simulink model "PassiveHydPTO_Version_2"  (R2014a)
settings: Solver=ode23tb  StartTime=0.0  StopTime=param.stop  FixedStep=0.01  MaxStep=0.05  RelTol=1e-6
values from neighbouring files (symbols this model uses):
  alpha = 1    [Main.m]
  Amax = 0.001    [Main.m]
  Amin = 1e-8    (= 1e-08)    [Main.m]
  Ap = 2.35e-2    (= 0.0235)    [Main.m]
  Beta_e = 1.86e9    (= 1860000000)    [Main.m]
  bf = 0.05*bg    (= 0.118735)    [Main.m]
  bg = 2.3747    [Main.m]
  Cd = 0.61    [Main.m]
  D = 3.9789e-5    (= 3.9789e-05)    [Main.m]
  Dh = sqrt(4*Av/pi)    [Main.m]
  f = 1/period    (= 0.1)    [Main.m]
  J = 3.961    [Main.m]
  k1 = 200    [Main.m]
  k2 = atanh((Amin-(Amax-Amin)/2)*      2/(Amax - Amin))*1/(pMin-(pMax + pMin)/2)    [Main.m]
  omega_i = 0    [Main.m]
  pAeq = pCeq    (= 21333333.3333)    [Main.m]
  pAi = pAeq    (= 21333333.3333)    [Main.m]
  pAupper_limit = 32e6    (= 32000000)    [Main.m]
  pBeq = pCeq    (= 21333333.3333)    [Main.m]
  pBi = pBeq    (= 21333333.3333)    [Main.m]
  pBupper_limit = 32e6    (= 32000000)    [Main.m]
  pCprecharge = 0.9*pClower_limit    (= 19200000)    [Main.m]
  pDprecharge = 0.9*pDlower_limit    (= 9600000)    [Main.m]
  pMax = 1e6    (= 1000000)    [Main.m]
  pMin = 0.75e6    (= 750000)    [Main.m]
  rho = 850    [Main.m]
  Rt = 10    [Main.m]
  v = 5.5e-5    (= 5.5e-05)    [Main.m]
  VC0 = 7.5    [Main.m]
  VCeq = VC0*(1-(pCprecharge/pCeq)^(1/1.4))    (= 0.543715404282)    [Main.m]
  VD0 = 3    [Main.m]
  VDeq = VDmax    (= 1.30403881906)    [Main.m]
  Vo = Ap*5    (= 0.1175)    [Main.m]
undefined symbols (not defined in the file or in its folder): magnitude
settings Model: Creator=sor  LastModifiedBy=sor

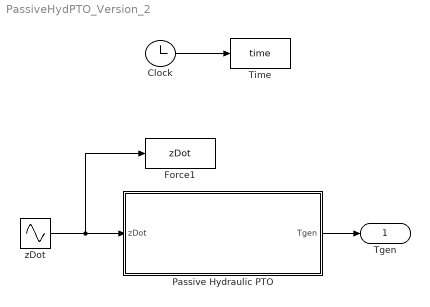
== system PassiveHydPTO_Version_2 ==
  Clock : Clock
  Force1 : ToWorkspace  VariableName=zDot  SampleTime=-1
  "Passive Hydraulic PTO " : Subsystem
  Time : ToWorkspace  VariableName=time  SampleTime=-1
  zDot : Sin  Amplitude=0.8  Frequency=2*pi*f  SampleTime=0
  Tgen : Outport
  wires:
  Clock/1 -> Time/1
  zDot/1 -> Force1/1, "Passive Hydraulic PTO "/1(zDot)
  "Passive Hydraulic PTO "/1(Tgen) -> Tgen/1

== system PassiveHydPTO_Version_2/Passive Hydraulic PTO  ==
  zDot : Inport
  High Pressure Accumulator : Subsystem
  Low Pressure Accumulator : Subsystem
  Motor Generator : Subsystem
  "Piston Pump " : Subsystem
  Rectified Valve : Subsystem
  Tgen : Outport
  wires:
  "Piston Pump "/1(pA) -> Rectified Valve/1(pA)
  Motor Generator/1(Tgen) -> Tgen/1
  Rectified Valve/1(Vdot1) -> High Pressure Accumulator/1(Vdot1)
  Rectified Valve/2(Vdot2) -> High Pressure Accumulator/2(Vdot2)
  Rectified Valve/3(Vdot3) -> Low Pressure Accumulator/1(Vdot3)
  Rectified Valve/4(Vdot4) -> Low Pressure Accumulator/2(Vdot4)
  High Pressure Accumulator/1(pC) -> Motor Generator/1(pC)
  Low Pressure Accumulator/1(pD) -> Motor Generator/2(pD)
  "Piston Pump "/2(pB) -> Rectified Valve/2(pB)
  zDot/1 -> "Piston Pump "/1(zDot)

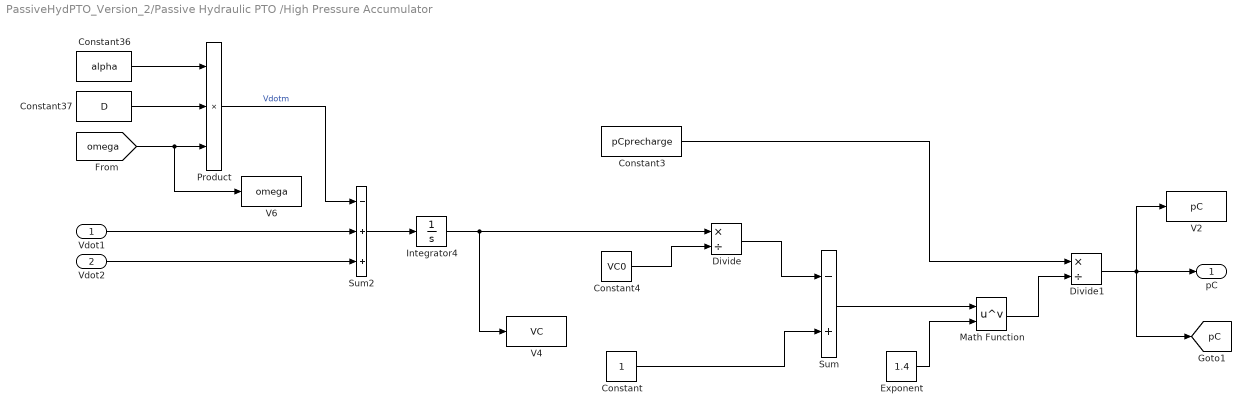
== system PassiveHydPTO_Version_2/Passive Hydraulic PTO /High Pressure Accumulator ==
  Vdot1 : Inport
  Vdot2 : Inport  Port=2
  Constant : Constant
  Constant3 : Constant  Value=pCprecharge
  Constant36 : Constant  Value=alpha
  Constant37 : Constant  Value=D
  Constant4 : Constant  Value=VC0
  Divide : Product  Inputs=*/
  Divide1 : Product  Inputs=*/
  Exponent : Constant  Value=1.4
  Integrator4 : Integrator  InitialCondition=VCeq
  Math Function : Math  Operator=pow  SaturateOnIntegerOverflow=on
  Product : Product  Inputs=3
  Sum : Sum  Inputs=-+
  Sum2 : Sum  Inputs=-++
  V2 : ToWorkspace  VariableName=pC  SampleTime=-1
  V4 : ToWorkspace  VariableName=VC  SampleTime=-1
  V6 : ToWorkspace  VariableName=omega  SampleTime=-1
  pC : Outport
  tag scope: pC=global
  wires:
  Constant36/1 -> Product/1
  Constant37/1 -> Product/2
  [omega] -> V6/1, Product/3
  Product/1 -> Sum2/1  "Vdotm"
  Vdot1/1 -> Sum2/2
  Vdot2/1 -> Sum2/3
  Sum2/1 -> Integrator4/1
  Integrator4/1 -> Divide/1, V4/1
  Constant4/1 -> Divide/2
  Constant/1 -> Sum/2
  Divide/1 -> Sum/1
  Exponent/1 -> Math Function/2
  Sum/1 -> Math Function/1
  Math Function/1 -> Divide1/2
  Constant3/1 -> Divide1/1
  Divide1/1 -> [pC], V2/1, pC/1

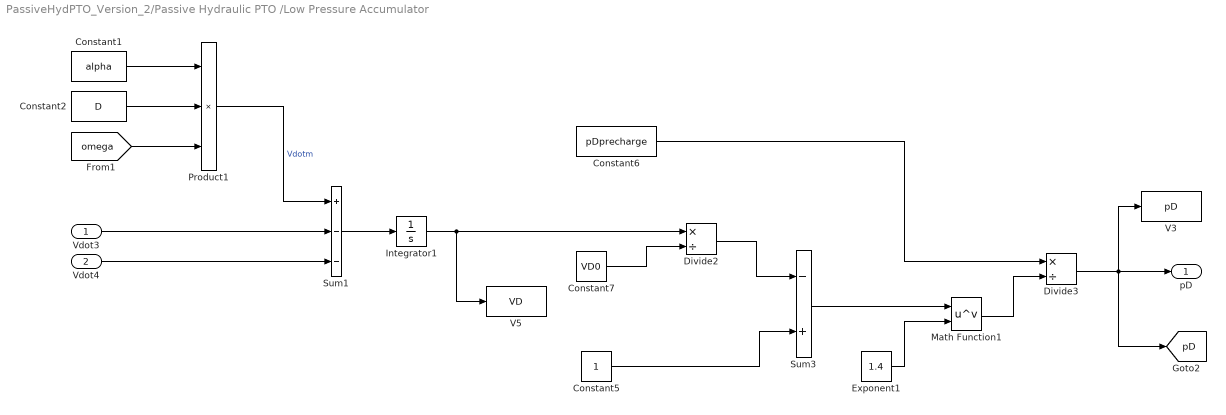
== system PassiveHydPTO_Version_2/Passive Hydraulic PTO /Low Pressure Accumulator ==
  Vdot3 : Inport
  Vdot4 : Inport  Port=2
  Constant1 : Constant  Value=alpha
  Constant2 : Constant  Value=D
  Constant5 : Constant
  Constant6 : Constant  Value=pDprecharge
  Constant7 : Constant  Value=VD0
  Divide2 : Product  Inputs=*/
  Divide3 : Product  Inputs=*/
  Exponent1 : Constant  Value=1.4
  Integrator1 : Integrator  InitialCondition=VDeq
  Math Function1 : Math  Operator=pow  SaturateOnIntegerOverflow=on
  Product1 : Product  Inputs=3
  Sum1 : Sum  Inputs=+--
  Sum3 : Sum  Inputs=-+
  V3 : ToWorkspace  VariableName=pD  SampleTime=-1
  V5 : ToWorkspace  VariableName=VD  SampleTime=-1
  pD : Outport
  tag scope: pD=global
  wires:
  Constant1/1 -> Product1/1
  Constant2/1 -> Product1/2
  [omega] -> Product1/3
  Product1/1 -> Sum1/1  "Vdotm"
  Vdot3/1 -> Sum1/2
  Vdot4/1 -> Sum1/3
  Sum1/1 -> Integrator1/1
  Integrator1/1 -> Divide2/1, V5/1
  Constant7/1 -> Divide2/2
  Constant5/1 -> Sum3/2
  Divide2/1 -> Sum3/1
  Exponent1/1 -> Math Function1/2
  Sum3/1 -> Math Function1/1
  Math Function1/1 -> Divide3/2
  Constant6/1 -> Divide3/1
  Divide3/1 -> [pD], V3/1, pD/1

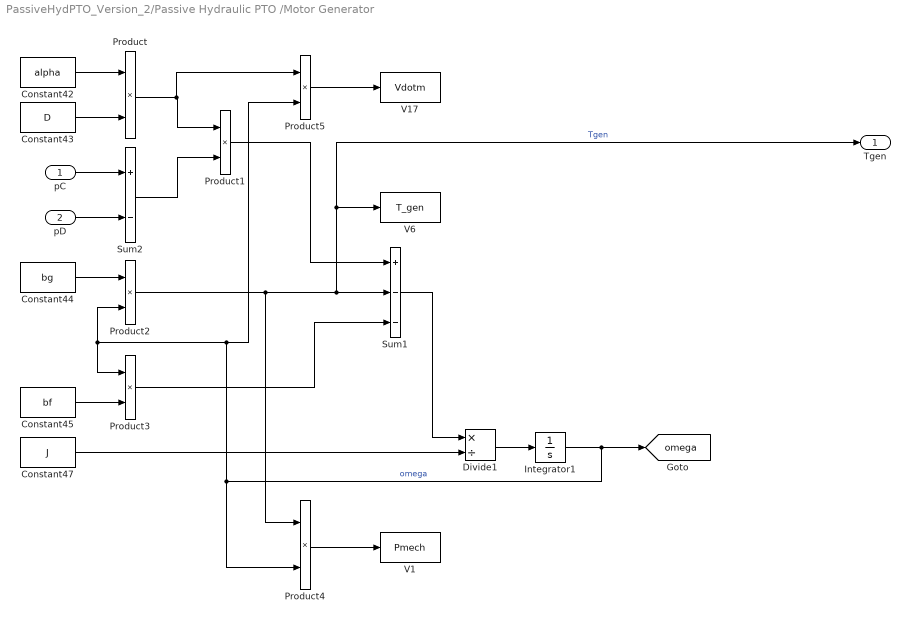
== system PassiveHydPTO_Version_2/Passive Hydraulic PTO /Motor Generator ==
  pC : Inport
  pD : Inport  Port=2
  Constant42 : Constant  Value=alpha
  Constant43 : Constant  Value=D
  Constant44 : Constant  Value=bg
  Constant45 : Constant  Value=bf
  Constant47 : Constant  Value=J
  Divide1 : Product  Inputs=*/
  Integrator1 : Integrator  InitialCondition=omega_i
  Product{,1..5} (6 alike) : Product
  Sum1 : Sum  Inputs=+--
  Sum2 : Sum  Inputs=+-
  V1 : ToWorkspace  VariableName=Pmech  SampleTime=-1
  V17 : ToWorkspace  VariableName=Vdotm  SampleTime=-1
  V6 : ToWorkspace  VariableName=T_gen  SampleTime=-1
  Tgen : Outport
  tag scope: omega=global
  wires:
  Constant42/1 -> Product/1
  Constant43/1 -> Product/2
  pC/1 -> Sum2/1
  pD/1 -> Sum2/2
  Product/1 -> Product5/1, Product1/1
  Sum2/1 -> Product1/2
  Constant44/1 -> Product2/1
  Constant45/1 -> Product3/2
  Product1/1 -> Sum1/1
  Product2/1 -> Product4/1, Tgen/1, V6/1, Sum1/2  "Tgen"
  Product3/1 -> Sum1/3
  Sum1/1 -> Divide1/1
  Constant47/1 -> Divide1/2
  Product4/1 -> V1/1
  Divide1/1 -> Integrator1/1
  Integrator1/1 -> Product4/2, Product3/1, Product2/2, Product5/2, [omega]  "omega"
  Product5/1 -> V17/1

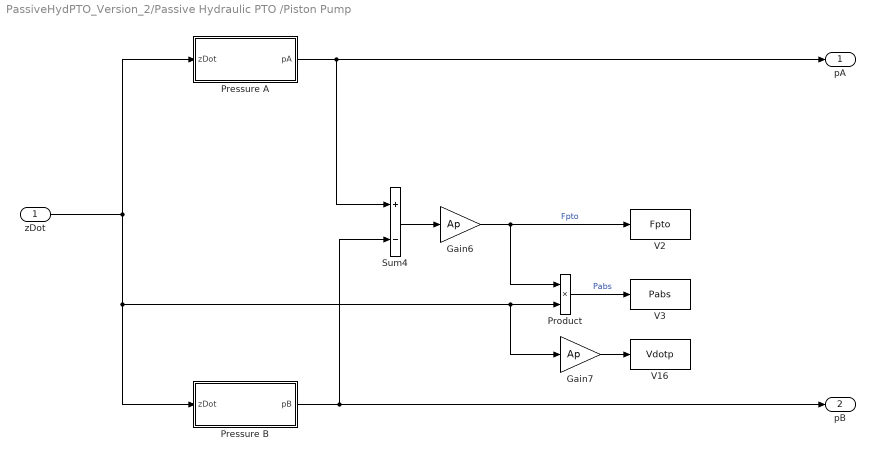
== system PassiveHydPTO_Version_2/Passive Hydraulic PTO /Piston Pump  ==
  zDot : Inport
  Gain6 : Gain  Gain=Ap
  Gain7 : Gain  Gain=Ap
  Pressure A : Subsystem
  Pressure B : Subsystem
  Product : Product
  Sum4 : Sum  Inputs=+-
  V16 : ToWorkspace  VariableName=Vdotp  SampleTime=-1
  V2 : ToWorkspace  VariableName=Fpto  SampleTime=-1
  V3 : ToWorkspace  VariableName=Pabs  SampleTime=-1
  pA : Outport
  pB : Outport  Port=2
  wires:
  zDot/1 -> Pressure A/1(zDot), Gain7/1, Product/2, Pressure B/1(zDot)
  Pressure A/1(pA) -> pA/1, Sum4/1
  Pressure B/1(pB) -> Sum4/2, pB/1
  Sum4/1 -> Gain6/1
  Gain7/1 -> V16/1
  Gain6/1 -> V2/1, Product/1  "Fpto"
  Product/1 -> V3/1  "Pabs"

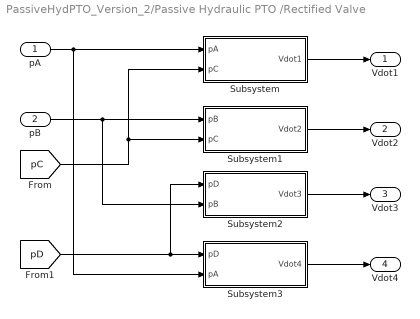
== system PassiveHydPTO_Version_2/Passive Hydraulic PTO /Rectified Valve ==
  pA : Inport
  pB : Inport  Port=2
  Subsystem : Subsystem
  Subsystem1 : Subsystem
  Subsystem2 : Subsystem
  Subsystem3 : Subsystem
  Vdot1 : Outport
  Vdot2 : Outport  Port=2
  Vdot3 : Outport  Port=3
  Vdot4 : Outport  Port=4
  wires:
  pA/1 -> Subsystem/1(pA), Subsystem3/2(pA)
  pB/1 -> Subsystem2/2(pB), Subsystem1/1(pB)
  [pC] -> Subsystem1/2(pC), Subsystem/2(pC)
  [pD] -> Subsystem3/1(pD), Subsystem2/1(pD)
  Subsystem3/1(Vdot4) -> Vdot4/1
  Subsystem2/1(Vdot3) -> Vdot3/1
  Subsystem1/1(Vdot2) -> Vdot2/1
  Subsystem/1(Vdot1) -> Vdot1/1

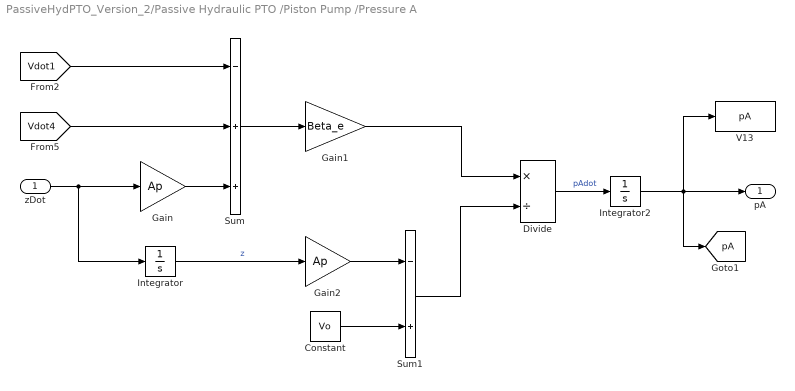
== system PassiveHydPTO_Version_2/Passive Hydraulic PTO /Piston Pump /Pressure A ==
  zDot : Inport
  Constant : Constant  Value=Vo
  Divide : Product  Inputs=*/
  Gain : Gain  Gain=Ap
  Gain1 : Gain  Gain=Beta_e
  Gain2 : Gain  Gain=Ap
  Integrator : Integrator
  Integrator2 : Integrator  InitialCondition=pAi  UpperSaturationLimit=pAupper_limit  LowerSaturationLimit=pAeq
  Sum : Sum  Inputs=-++
  Sum1 : Sum  Inputs=-+
  V13 : ToWorkspace  VariableName=pA  SampleTime=-1
  pA : Outport
  tag scope: pA=global
  wires:
  Gain/1 -> Sum/3
  Sum/1 -> Gain1/1
  zDot/1 -> Integrator/1, Gain/1
  Integrator/1 -> Gain2/1  "z"
  Gain2/1 -> Sum1/1
  Constant/1 -> Sum1/2
  Gain1/1 -> Divide/1
  Sum1/1 -> Divide/2
  [Vdot1] -> Sum/1
  Divide/1 -> Integrator2/1  "pAdot"
  [Vdot4] -> Sum/2
  Integrator2/1 -> pA/1, [pA], V13/1

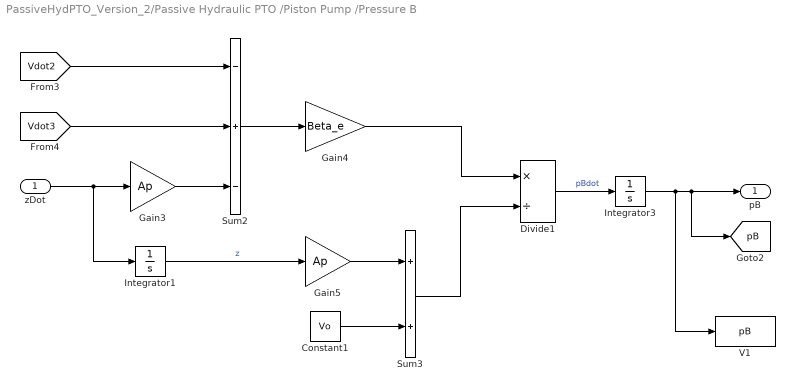
== system PassiveHydPTO_Version_2/Passive Hydraulic PTO /Piston Pump /Pressure B ==
  zDot : Inport
  Constant1 : Constant  Value=Vo
  Divide1 : Product  Inputs=*/
  Gain3 : Gain  Gain=Ap
  Gain4 : Gain  Gain=Beta_e
  Gain5 : Gain  Gain=Ap
  Integrator1 : Integrator
  Integrator3 : Integrator  InitialCondition=pBi  UpperSaturationLimit=pBupper_limit  LowerSaturationLimit=pBeq
  Sum2 : Sum  Inputs=-+-
  Sum3 : Sum
  V1 : ToWorkspace  VariableName=pB  SampleTime=-1
  pB : Outport
  tag scope: pB=global
  wires:
  Gain3/1 -> Sum2/3
  Sum2/1 -> Gain4/1
  zDot/1 -> Integrator1/1, Gain3/1
  Integrator1/1 -> Gain5/1  "z"
  Gain5/1 -> Sum3/1
  Constant1/1 -> Sum3/2
  Gain4/1 -> Divide1/1
  Sum3/1 -> Divide1/2
  Divide1/1 -> Integrator3/1  "pBdot"
  [Vdot2] -> Sum2/1
  [Vdot3] -> Sum2/2
  Integrator3/1 -> V1/1, pB/1, [pB]

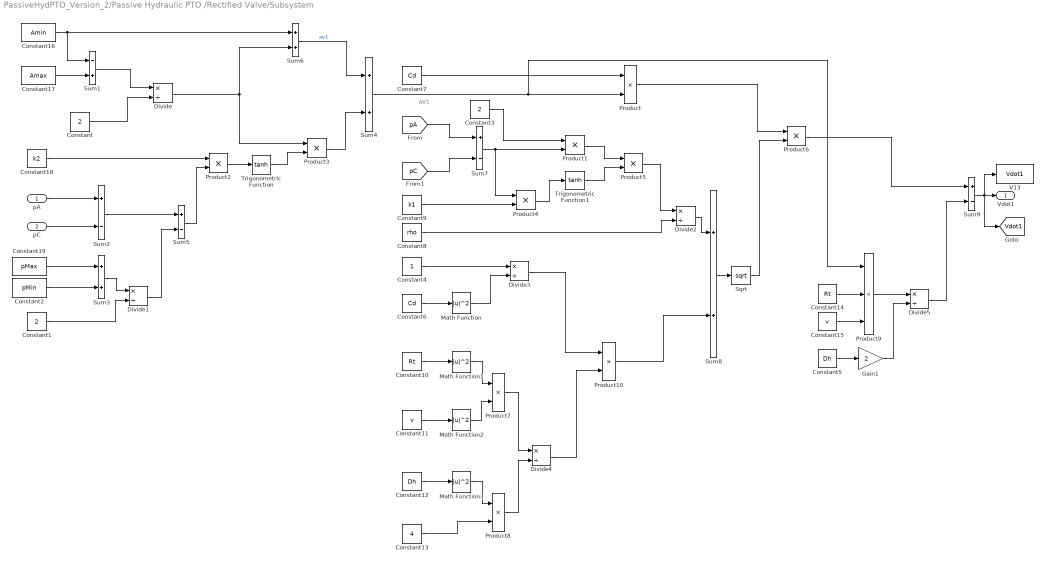
== system PassiveHydPTO_Version_2/Passive Hydraulic PTO /Rectified Valve/Subsystem ==
  note: aV1
  pA : Inport
  pC : Inport  Port=2
  Constant : Constant  Value=2
  Constant1 : Constant  Value=2
  Constant10 : Constant  Value=Rt
  Constant11 : Constant  Value=v
  Constant12 : Constant  Value=Dh
  Constant13 : Constant  Value=4
  Constant14 : Constant  Value=Rt
  Constant15 : Constant  Value=v
  Constant16 : Constant  Value=Amin
  Constant17 : Constant  Value=Amax
  Constant18 : Constant  Value=k2
  Constant19 : Constant  Value=pMax
  Constant2 : Constant  Value=pMin
  Constant3 : Constant  Value=2
  Constant4 : Constant
  Constant5 : Constant  Value=Dh
  Constant6 : Constant  Value=Cd
  Constant7 : Constant  Value=Cd
  Constant8 : Constant  Value=rho
  Constant9 : Constant  Value=k1
  Divide{,1..5} (6 alike) : Product  Inputs=*/
  Gain1 : Gain  Gain=2
  Math Function{,1..3} (4 alike) : Math  Operator=magnitude^2  SaturateOnIntegerOverflow=on
  Product{,1..8,10} (10 alike) : Product
  Product9 : Product  Inputs=3
  Sqrt : Sqrt  SaturateOnIntegerOverflow=on
  Sum1 : Sum  Inputs=-+
  Sum{2,5,7,9} (4 alike) : Sum  Inputs=+-
  Sum{3..4,6,8} (4 alike) : Sum
  Trigonometric Function : Trigonometry  Operator=tanh
  Trigonometric Function1 : Trigonometry  Operator=tanh
  V13 : ToWorkspace  VariableName=Vdot1  SampleTime=-1
  Vdot1 : Outport
  tag scope: Vdot1=global
  wires:
  Constant16/1 -> Sum6/1, Sum1/1
  Constant17/1 -> Sum1/2
  Sum1/1 -> Divide/1
  Constant/1 -> Divide/2
  Product2/1 -> Trigonometric Function/1
  Trigonometric Function/1 -> Product3/2
  Product3/1 -> Sum4/2
  pA/1 -> Sum2/1
  Constant19/1 -> Sum3/1
  Constant2/1 -> Sum3/2
  Sum3/1 -> Divide1/1
  Constant1/1 -> Divide1/2
  Divide/1 -> Sum6/2, Product3/1
  Sum2/1 -> Sum5/1
  Divide1/1 -> Sum5/2
  Constant18/1 -> Product2/1
  Sum5/1 -> Product2/2
  Sum6/1 -> Sum4/1  "av1"
  pC/1 -> Sum2/2
  Constant7/1 -> Product/1
  Sum4/1 -> Product9/1, Product/2
  Sum7/1 -> Product4/1, Product1/2
  Constant3/1 -> Product1/1
  Constant9/1 -> Product4/2
  Product4/1 -> Trigonometric Function1/1
  Product1/1 -> Product5/1
  Trigonometric Function1/1 -> Product5/2
  Sqrt/1 -> Product6/2
  Product/1 -> Product6/1
  Constant8/1 -> Divide2/2
  Product5/1 -> Divide2/1
  Divide2/1 -> Sum8/1
  Sum8/1 -> Sqrt/1
  Product6/1 -> Sum9/1
  Constant14/1 -> Product9/2
  Constant15/1 -> Product9/3
  Product9/1 -> Divide5/1
  Constant5/1 -> Gain1/1
  Gain1/1 -> Divide5/2
  Divide5/1 -> Sum9/2
  Product10/1 -> Sum8/2
  Constant4/1 -> Divide3/1
  Constant6/1 -> Math Function/1
  Math Function/1 -> Divide3/2
  Constant10/1 -> Math Function1/1
  Constant11/1 -> Math Function2/1
  Math Function1/1 -> Product7/1
  Math Function2/1 -> Product7/2
  Constant12/1 -> Math Function3/1
  Math Function3/1 -> Product8/1
  Constant13/1 -> Product8/2
  Product7/1 -> Divide4/1
  Product8/1 -> Divide4/2
  Divide3/1 -> Product10/1
  Divide4/1 -> Product10/2
  [pA] -> Sum7/1
  [pC] -> Sum7/2
  Sum9/1 -> [Vdot1], V13/1, Vdot1/1

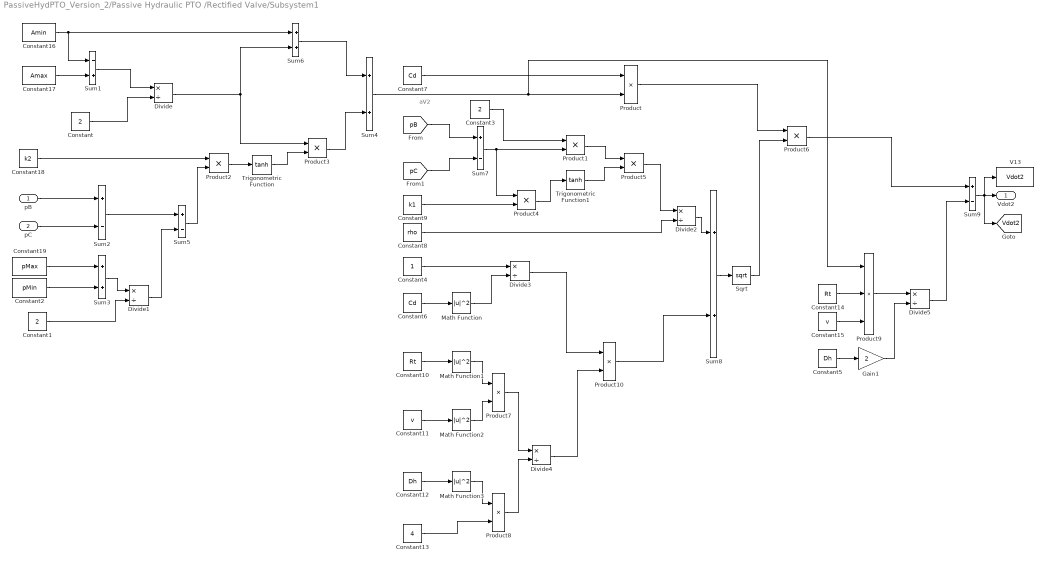
== system PassiveHydPTO_Version_2/Passive Hydraulic PTO /Rectified Valve/Subsystem1 ==
  note: aV2
  pB : Inport
  pC : Inport  Port=2
  Constant : Constant  Value=2
  Constant1 : Constant  Value=2
  Constant10 : Constant  Value=Rt
  Constant11 : Constant  Value=v
  Constant12 : Constant  Value=Dh
  Constant13 : Constant  Value=4
  Constant14 : Constant  Value=Rt
  Constant15 : Constant  Value=v
  Constant16 : Constant  Value=Amin
  Constant17 : Constant  Value=Amax
  Constant18 : Constant  Value=k2
  Constant19 : Constant  Value=pMax
  Constant2 : Constant  Value=pMin
  Constant3 : Constant  Value=2
  Constant4 : Constant
  Constant5 : Constant  Value=Dh
  Constant6 : Constant  Value=Cd
  Constant7 : Constant  Value=Cd
  Constant8 : Constant  Value=rho
  Constant9 : Constant  Value=k1
  Divide{,1..5} (6 alike) : Product  Inputs=*/
  Gain1 : Gain  Gain=2
  Math Function{,1..3} (4 alike) : Math  Operator=magnitude^2  SaturateOnIntegerOverflow=on
  Product{,1..8,10} (10 alike) : Product
  Product9 : Product  Inputs=3
  Sqrt : Sqrt  SaturateOnIntegerOverflow=on
  Sum1 : Sum  Inputs=-+
  Sum{2,5,7,9} (4 alike) : Sum  Inputs=+-
  Sum{3..4,6,8} (4 alike) : Sum
  Trigonometric Function : Trigonometry  Operator=tanh
  Trigonometric Function1 : Trigonometry  Operator=tanh
  V13 : ToWorkspace  VariableName=Vdot2  SampleTime=-1
  Vdot2 : Outport
  tag scope: Vdot2=global
  wires:
  Constant16/1 -> Sum6/1, Sum1/1
  Constant17/1 -> Sum1/2
  Sum1/1 -> Divide/1
  Constant/1 -> Divide/2
  Product2/1 -> Trigonometric Function/1
  Trigonometric Function/1 -> Product3/2
  Product3/1 -> Sum4/2
  pB/1 -> Sum2/1
  Constant19/1 -> Sum3/1
  Constant2/1 -> Sum3/2
  Sum3/1 -> Divide1/1
  Constant1/1 -> Divide1/2
  Divide/1 -> Sum6/2, Product3/1
  Sum2/1 -> Sum5/1
  Divide1/1 -> Sum5/2
  Constant18/1 -> Product2/1
  Sum5/1 -> Product2/2
  Sum6/1 -> Sum4/1
  pC/1 -> Sum2/2
  Constant7/1 -> Product/1
  Sum4/1 -> Product9/1, Product/2
  Sum7/1 -> Product4/1, Product1/2
  Constant3/1 -> Product1/1
  Constant9/1 -> Product4/2
  Product4/1 -> Trigonometric Function1/1
  Product1/1 -> Product5/1
  Trigonometric Function1/1 -> Product5/2
  Sqrt/1 -> Product6/2
  Product/1 -> Product6/1
  Constant8/1 -> Divide2/2
  Product5/1 -> Divide2/1
  Divide2/1 -> Sum8/1
  Sum8/1 -> Sqrt/1
  Product6/1 -> Sum9/1
  Constant14/1 -> Product9/2
  Constant15/1 -> Product9/3
  Product9/1 -> Divide5/1
  Constant5/1 -> Gain1/1
  Gain1/1 -> Divide5/2
  Divide5/1 -> Sum9/2
  Product10/1 -> Sum8/2
  Constant4/1 -> Divide3/1
  Constant6/1 -> Math Function/1
  Math Function/1 -> Divide3/2
  Constant10/1 -> Math Function1/1
  Constant11/1 -> Math Function2/1
  Math Function1/1 -> Product7/1
  Math Function2/1 -> Product7/2
  Constant12/1 -> Math Function3/1
  Math Function3/1 -> Product8/1
  Constant13/1 -> Product8/2
  Product7/1 -> Divide4/1
  Product8/1 -> Divide4/2
  Divide3/1 -> Product10/1
  Divide4/1 -> Product10/2
  [pB] -> Sum7/1
  [pC] -> Sum7/2
  Sum9/1 -> [Vdot2], V13/1, Vdot2/1

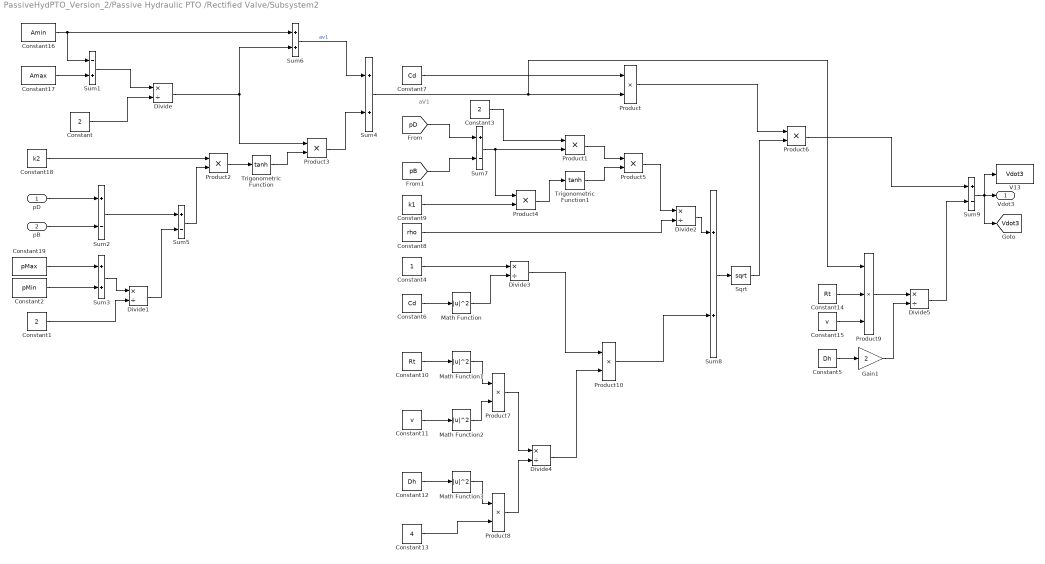
== system PassiveHydPTO_Version_2/Passive Hydraulic PTO /Rectified Valve/Subsystem2 ==
  note: aV1
  pD : Inport
  pB : Inport  Port=2
  Constant : Constant  Value=2
  Constant1 : Constant  Value=2
  Constant10 : Constant  Value=Rt
  Constant11 : Constant  Value=v
  Constant12 : Constant  Value=Dh
  Constant13 : Constant  Value=4
  Constant14 : Constant  Value=Rt
  Constant15 : Constant  Value=v
  Constant16 : Constant  Value=Amin
  Constant17 : Constant  Value=Amax
  Constant18 : Constant  Value=k2
  Constant19 : Constant  Value=pMax
  Constant2 : Constant  Value=pMin
  Constant3 : Constant  Value=2
  Constant4 : Constant
  Constant5 : Constant  Value=Dh
  Constant6 : Constant  Value=Cd
  Constant7 : Constant  Value=Cd
  Constant8 : Constant  Value=rho
  Constant9 : Constant  Value=k1
  Divide{,1..5} (6 alike) : Product  Inputs=*/
  Gain1 : Gain  Gain=2
  Math Function{,1..3} (4 alike) : Math  Operator=magnitude^2  SaturateOnIntegerOverflow=on
  Product{,1..8,10} (10 alike) : Product
  Product9 : Product  Inputs=3
  Sqrt : Sqrt  SaturateOnIntegerOverflow=on
  Sum1 : Sum  Inputs=-+
  Sum{2,5,7,9} (4 alike) : Sum  Inputs=+-
  Sum{3..4,6,8} (4 alike) : Sum
  Trigonometric Function : Trigonometry  Operator=tanh
  Trigonometric Function1 : Trigonometry  Operator=tanh
  V13 : ToWorkspace  VariableName=Vdot3  SampleTime=-1
  Vdot3 : Outport
  tag scope: Vdot3=global
  wires:
  Constant16/1 -> Sum6/1, Sum1/1
  Constant17/1 -> Sum1/2
  Sum1/1 -> Divide/1
  Constant/1 -> Divide/2
  Product2/1 -> Trigonometric Function/1
  Trigonometric Function/1 -> Product3/2
  Product3/1 -> Sum4/2
  pD/1 -> Sum2/1
  Constant19/1 -> Sum3/1
  Constant2/1 -> Sum3/2
  Sum3/1 -> Divide1/1
  Constant1/1 -> Divide1/2
  Divide/1 -> Sum6/2, Product3/1
  Sum2/1 -> Sum5/1
  Divide1/1 -> Sum5/2
  Constant18/1 -> Product2/1
  Sum5/1 -> Product2/2
  Sum6/1 -> Sum4/1  "av1"
  pB/1 -> Sum2/2
  Constant7/1 -> Product/1
  Sum4/1 -> Product9/1, Product/2
  Sum7/1 -> Product4/1, Product1/2
  Constant3/1 -> Product1/1
  Constant9/1 -> Product4/2
  Product4/1 -> Trigonometric Function1/1
  Product1/1 -> Product5/1
  Trigonometric Function1/1 -> Product5/2
  Sqrt/1 -> Product6/2
  Product/1 -> Product6/1
  Constant8/1 -> Divide2/2
  Product5/1 -> Divide2/1
  Divide2/1 -> Sum8/1
  Sum8/1 -> Sqrt/1
  Product6/1 -> Sum9/1
  Constant14/1 -> Product9/2
  Constant15/1 -> Product9/3
  Product9/1 -> Divide5/1
  Constant5/1 -> Gain1/1
  Gain1/1 -> Divide5/2
  Divide5/1 -> Sum9/2
  Product10/1 -> Sum8/2
  Constant4/1 -> Divide3/1
  Constant6/1 -> Math Function/1
  Math Function/1 -> Divide3/2
  Constant10/1 -> Math Function1/1
  Constant11/1 -> Math Function2/1
  Math Function1/1 -> Product7/1
  Math Function2/1 -> Product7/2
  Constant12/1 -> Math Function3/1
  Math Function3/1 -> Product8/1
  Constant13/1 -> Product8/2
  Product7/1 -> Divide4/1
  Product8/1 -> Divide4/2
  Divide3/1 -> Product10/1
  Divide4/1 -> Product10/2
  [pD] -> Sum7/1
  [pB] -> Sum7/2
  Sum9/1 -> [Vdot3], V13/1, Vdot3/1

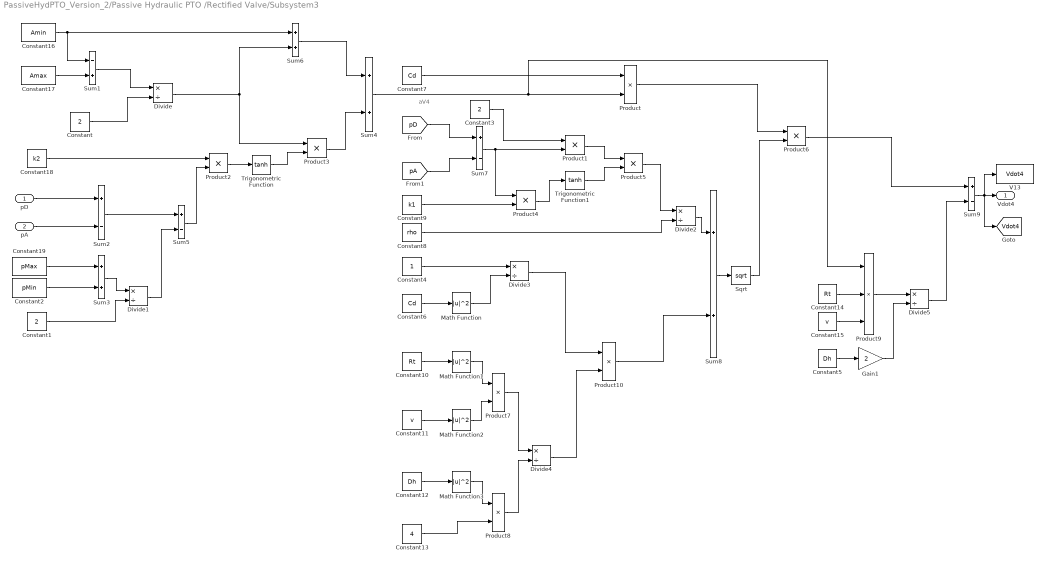
== system PassiveHydPTO_Version_2/Passive Hydraulic PTO /Rectified Valve/Subsystem3 ==
  note: aV4
  pD : Inport
  pA : Inport  Port=2
  Constant : Constant  Value=2
  Constant1 : Constant  Value=2
  Constant10 : Constant  Value=Rt
  Constant11 : Constant  Value=v
  Constant12 : Constant  Value=Dh
  Constant13 : Constant  Value=4
  Constant14 : Constant  Value=Rt
  Constant15 : Constant  Value=v
  Constant16 : Constant  Value=Amin
  Constant17 : Constant  Value=Amax
  Constant18 : Constant  Value=k2
  Constant19 : Constant  Value=pMax
  Constant2 : Constant  Value=pMin
  Constant3 : Constant  Value=2
  Constant4 : Constant
  Constant5 : Constant  Value=Dh
  Constant6 : Constant  Value=Cd
  Constant7 : Constant  Value=Cd
  Constant8 : Constant  Value=rho
  Constant9 : Constant  Value=k1
  Divide{,1..5} (6 alike) : Product  Inputs=*/
  Gain1 : Gain  Gain=2
  Math Function{,1..3} (4 alike) : Math  Operator=magnitude^2  SaturateOnIntegerOverflow=on
  Product{,1..8,10} (10 alike) : Product
  Product9 : Product  Inputs=3
  Sqrt : Sqrt  SaturateOnIntegerOverflow=on
  Sum1 : Sum  Inputs=-+
  Sum{2,5,7,9} (4 alike) : Sum  Inputs=+-
  Sum{3..4,6,8} (4 alike) : Sum
  Trigonometric Function : Trigonometry  Operator=tanh
  Trigonometric Function1 : Trigonometry  Operator=tanh
  V13 : ToWorkspace  VariableName=Vdot4  SampleTime=-1
  Vdot4 : Outport
  tag scope: Vdot4=global
  wires:
  Constant16/1 -> Sum6/1, Sum1/1
  Constant17/1 -> Sum1/2
  Sum1/1 -> Divide/1
  Constant/1 -> Divide/2
  Product2/1 -> Trigonometric Function/1
  Trigonometric Function/1 -> Product3/2
  Product3/1 -> Sum4/2
  pD/1 -> Sum2/1
  Constant19/1 -> Sum3/1
  Constant2/1 -> Sum3/2
  Sum3/1 -> Divide1/1
  Constant1/1 -> Divide1/2
  Divide/1 -> Sum6/2, Product3/1
  Sum2/1 -> Sum5/1
  Divide1/1 -> Sum5/2
  Constant18/1 -> Product2/1
  Sum5/1 -> Product2/2
  Sum6/1 -> Sum4/1
  pA/1 -> Sum2/2
  Constant7/1 -> Product/1
  Sum4/1 -> Product9/1, Product/2
  Sum7/1 -> Product4/1, Product1/2
  Constant3/1 -> Product1/1
  Constant9/1 -> Product4/2
  Product4/1 -> Trigonometric Function1/1
  Product1/1 -> Product5/1
  Trigonometric Function1/1 -> Product5/2
  Sqrt/1 -> Product6/2
  Product/1 -> Product6/1
  Constant8/1 -> Divide2/2
  Product5/1 -> Divide2/1
  Divide2/1 -> Sum8/1
  Sum8/1 -> Sqrt/1
  Product6/1 -> Sum9/1
  Constant14/1 -> Product9/2
  Constant15/1 -> Product9/3
  Product9/1 -> Divide5/1
  Constant5/1 -> Gain1/1
  Gain1/1 -> Divide5/2
  Divide5/1 -> Sum9/2
  Product10/1 -> Sum8/2
  Constant4/1 -> Divide3/1
  Constant6/1 -> Math Function/1
  Math Function/1 -> Divide3/2
  Constant10/1 -> Math Function1/1
  Constant11/1 -> Math Function2/1
  Math Function1/1 -> Product7/1
  Math Function2/1 -> Product7/2
  Constant12/1 -> Math Function3/1
  Math Function3/1 -> Product8/1
  Constant13/1 -> Product8/2
  Product7/1 -> Divide4/1
  Product8/1 -> Divide4/2
  Divide3/1 -> Product10/1
  Divide4/1 -> Product10/2
  [pD] -> Sum7/1
  [pA] -> Sum7/2
  Sum9/1 -> [Vdot4], V13/1, Vdot4/1
